simulink model "ejemplo2"  (R2025b)
settings: Solver=VariableStepAuto  StartTime=0.0  StopTime=10.0  RelTol=1e-3
settings DataIOCC: SaveFormat=Array  SaveState=on  SignalLogging=off  DSMLogging=off  ReturnWorkspaceOutputs=off

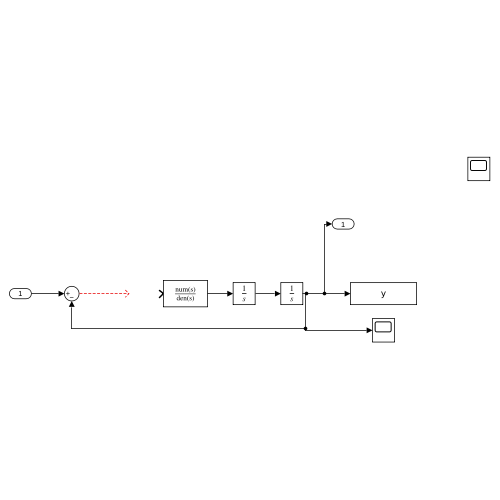
[thumbnail: Simulink's stored preview of the top-level diagram]
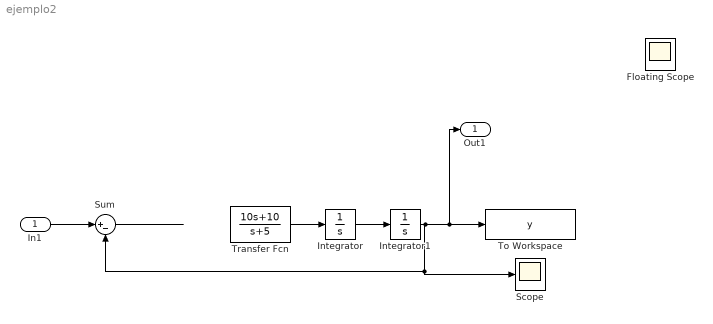
== system ejemplo2 ==
  In1 : Inport
  Floating Scope : Scope
      settings: IsFloating=on  Floating=on  ActiveDisplayYMinimum=-12.398784844335655  ActiveDisplayYMaximum=10.753715155664349
  Integrator : Integrator
  Integrator1 : Integrator
  Scope : Scope
  Sum : Sum  Inputs=|+-
  To Workspace : ToWorkspace  VariableName=y  SaveFormat=Timeseries  SampleTime=-1
  Transfer Fcn : TransferFcn  Numerator=[10 10]  Denominator=[1 5]
  Out1 : Outport
  wires:
  In1/1 -> Sum/1
  Sum/1 -> ?
  Transfer Fcn/1 -> Integrator/1
  Integrator/1 -> Integrator1/1
  Integrator1/1 -> To Workspace/1, Out1/1, Sum/2, Scope/1
